simulink model "QuarterCarModel"  (R2025b)
settings: Solver=VariableStepAuto  StartTime=0.0  StopTime=10.0  RelTol=1e-3
model workspace (MAT data in the model file):
  bs = 1500
  bt = 10
  ks = 20000
  kt = 190000
  ms = 400
  mu = 48
settings Model: Creator=khalidwaleed  LastModifiedBy=khalidwaleed

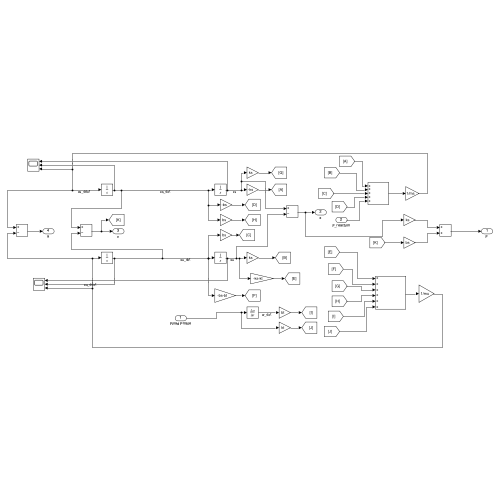
[thumbnail: Simulink's stored preview of the top-level diagram]
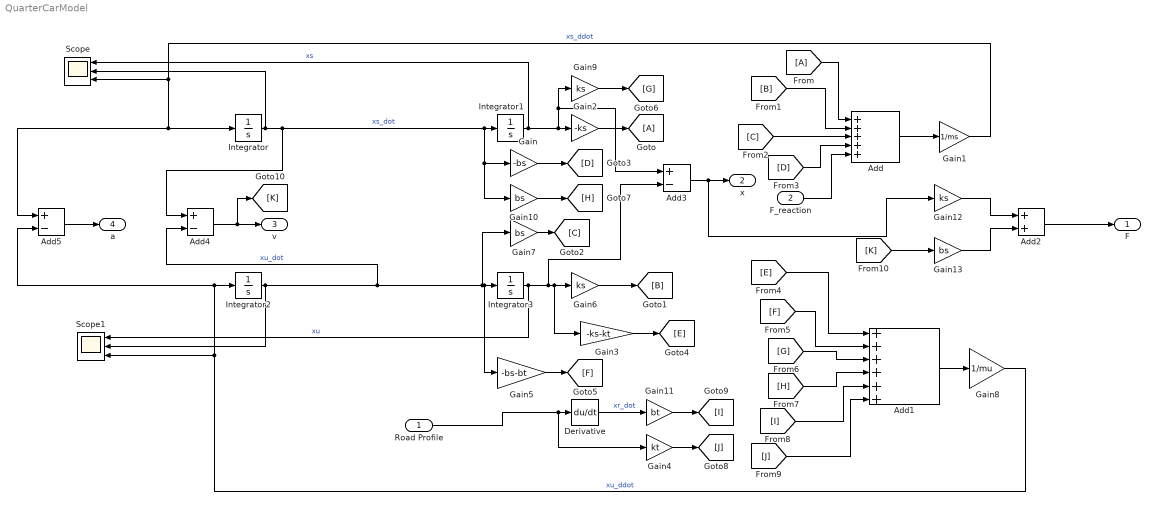
== system QuarterCarModel ==
  Road Profile : Inport
  F_reaction : Inport  Port=2  OutMin=[0.000000000000000001]  OutMax=[100000000000000000000000000]
  Add : Sum  Inputs=+++++
  Add1 : Sum  Inputs=++++++
  Add2 : Sum
  Add3 : Sum  Inputs=+-
  Add4 : Sum  Inputs=+-
  Add5 : Sum  Inputs=+-
  Derivative : Derivative
  From : From
  Gain : Gain  Gain=-bs
  Gain1 : Gain  Gain=1/ms
  Gain10 : Gain  Gain=bs
  Gain11 : Gain  Gain=bt
  Gain12 : Gain  Gain=ks
  Gain13 : Gain  Gain=bs
  Gain2 : Gain  Gain=-ks
  Gain3 : Gain  Gain=-ks-kt
  Gain4 : Gain  Gain=kt
  Gain5 : Gain  Gain=-bs-bt
  Gain6 : Gain  Gain=ks
  Gain7 : Gain  Gain=bs
  Gain8 : Gain  Gain=1/mu
  Gain9 : Gain  Gain=ks
  Goto : Goto
  Integrator{,1..3} (4 alike) : Integrator
  Scope : Scope  NumInputPorts=3
      settings: ActiveDisplayYMinimum=-4.4621453213775162  ActiveDisplayYMaximum=7.874735317035757
  Scope1 : Scope  NumInputPorts=3
      settings: ActiveDisplayYMinimum=-1  ActiveDisplayYMaximum=1
  F : Outport
  x : Outport  Port=2
  v : Outport  Port=3
  a : Outport  Port=4
  wires:
  Integrator2/1 -> Scope1/2, Add4/2, Gain7/1, Gain5/1, Integrator3/1  "xu_dot"
  Integrator/1 -> Scope/2, Add4/1, Gain10/1, Gain/1, Integrator1/1  "xs_dot"
  Gain1/1 -> Scope/3, Add5/1, Integrator/1  "xs_ddot"
  Integrator1/1 -> Scope/1, Gain9/1, Add3/1, Gain2/1  "xs"
  Gain8/1 -> Add5/2, Integrator2/1, Scope1/3  "xu_ddot"
  Integrator3/1 -> Scope1/1, Add3/2, Gain3/1, Gain6/1  "xu"
  Add/1 -> Gain1/1
  Add1/1 -> Gain8/1
  Derivative/1 -> Gain11/1  "xr_dot"
  Gain2/1 -> Goto/1
  From/1 -> Add/1
  Gain6/1 -> [B]
  [B] -> Add/2
  Gain7/1 -> [C]
  [C] -> Add/3
  Gain/1 -> [D]
  [D] -> Add/4
  Gain3/1 -> [E]
  [E] -> Add1/1
  Gain5/1 -> [F]
  [F] -> Add1/2
  Gain9/1 -> [G]
  [G] -> Add1/3
  Gain10/1 -> [H]
  [H] -> Add1/4
  [I] -> Add1/5
  [J] -> Add1/6
  Gain11/1 -> [I]
  Gain4/1 -> [J]
  Add2/1 -> F/1
  Add3/1 -> Gain12/1, x/1
  Add4/1 -> [K], v/1
  Add5/1 -> a/1
  [K] -> Gain13/1
  Gain12/1 -> Add2/1
  Gain13/1 -> Add2/2
  F_reaction/1 -> Add/5
  Road Profile/1 -> Gain4/1, Derivative/1
